simulink model "Boost_FLC_Current_State_Control"  (R2015b)
settings: Solver=ode23t  SolverMode=SingleTasking  StartTime=0.0  StopTime=0.1  FixedStep=1e-8  MinStep=1e-8  RelTol=1e-8
libraries: powerlib x8, fuzblock x2, powerlib_meascontrol x1
settings Model: Creator=Nady  LastModifiedBy=Nady
settings SolverCC: MaxConsecutiveMinStep=10  ZeroCrossAlgorithm=Adaptive  AlgebraicLoopSolver=LineSearch

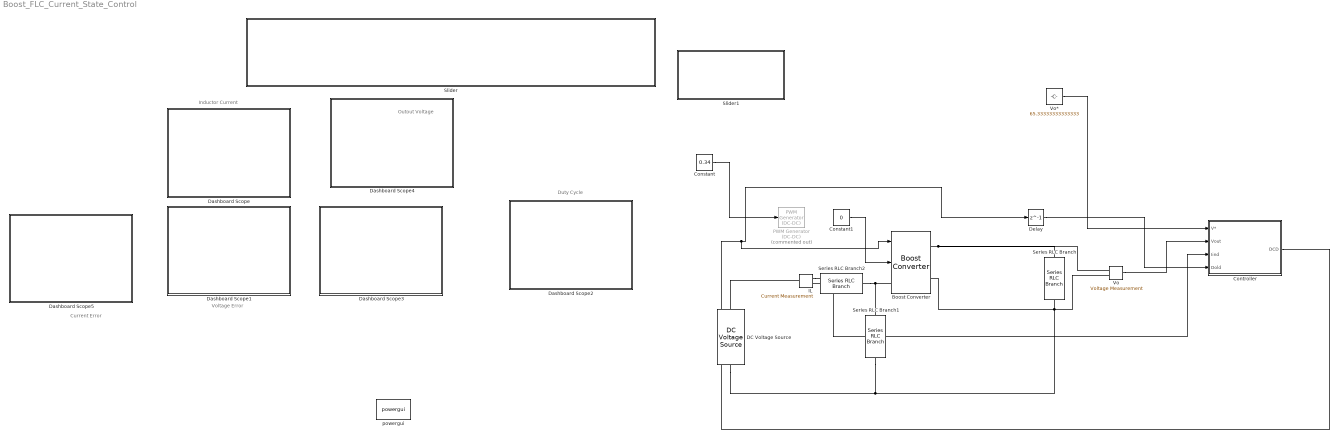
== system Boost_FLC_Current_State_Control ==
  note: Outout Voltage
  note: Inductor Current
  note: Current Error
  note: Duty Cycle
  note: Voltage Error
  Boost Converter : powerlib/Power Electronics/Boost Converter  ModelType=Average model (D-controlled)  Ron=1e-3  Rs=1e6  Cs=inf  Vforward=[0,0]  Ron_Diode=1e-3  Rs_Diode=1e6  Cs_Diode=inf  Vf_Diode=1e-3  Rs_CurrentSource=inf
  Constant : Constant  Value=0.34
  Constant1 : Constant  Value=0
  Controller : Subsystem  TreatAsAtomicUnit=on
  DC Voltage Source : powerlib/Electrical Sources/DC Voltage Source  Amplitude=50  Measurements=None
  Dashboard Scope : Subsystem  DialogController=hmiCreateDDGDialog  IsWebBlock=on  mask(MWDashboardBlock){webBlockId=b3b1b5ba-4a8f-4f28-bbe0-cb5b525e21d4, webBlockType=sdiscope, ShowInitialText=on, HMISrcModelName=Pilot_2_Sub_v4}
      mask prompts: webBlockId "WebBlock Id"; webBlockType "WebBlock Type"; HMISrcModelName "Source Model"
      mask Help: helpview([docroot '/mapfiles/simulink.map'], 'hmi_scope')
      mask Display:
      | if strcmp(get_param(bdroot(gcb),'BlockDiagramType'), 'library')
      |     image([(matlabroot) '/toolbox/simulink/hmi/icons/DashboardScope.png']);
      | end
  Dashboard Scope1 : Subsystem  DialogController=hmiCreateDDGDialog  IsWebBlock=on  mask(MWDashboardBlock){webBlockId=48ecfed1-8b3c-48bc-b34f-bf7039167704, webBlockType=sdiscope, ShowInitialText=on, HMISrcModelName=Pilot_2_Sub_v4}
      mask prompts: webBlockId "WebBlock Id"; webBlockType "WebBlock Type"; HMISrcModelName "Source Model"
      mask Help: helpview([docroot '/mapfiles/simulink.map'], 'hmi_scope')
      mask Display:
      | if strcmp(get_param(bdroot(gcb),'BlockDiagramType'), 'library')
      |     image([(matlabroot) '/toolbox/simulink/hmi/icons/DashboardScope.png']);
      | end
  Dashboard Scope2 : Subsystem  DialogController=hmiCreateDDGDialog  IsWebBlock=on  mask(MWDashboardBlock){webBlockId=b48e5165-dc27-41d1-8306-fea3cbfbff92, webBlockType=sdiscope, ShowInitialText=on, HMISrcModelName=Pilot_2_Sub_v4}
      mask prompts: webBlockId "WebBlock Id"; webBlockType "WebBlock Type"; HMISrcModelName "Source Model"
      mask Help: helpview([docroot '/mapfiles/simulink.map'], 'hmi_scope')
      mask Display:
      | if strcmp(get_param(bdroot(gcb),'BlockDiagramType'), 'library')
      |     image([(matlabroot) '/toolbox/simulink/hmi/icons/DashboardScope.png']);
      | end
  Dashboard Scope3 : Subsystem  DialogController=hmiCreateDDGDialog  IsWebBlock=on  mask(MWDashboardBlock){webBlockId=3429aff5-e82d-44ff-95e7-f1fb18ddd431, webBlockType=sdiscope, ShowInitialText=on, HMISrcModelName=Pilot_2_Sub_v4}
      mask prompts: webBlockId "WebBlock Id"; webBlockType "WebBlock Type"; HMISrcModelName "Source Model"
      mask Help: helpview([docroot '/mapfiles/simulink.map'], 'hmi_scope')
      mask Display:
      | if strcmp(get_param(bdroot(gcb),'BlockDiagramType'), 'library')
      |     image([(matlabroot) '/toolbox/simulink/hmi/icons/DashboardScope.png']);
      | end
  Dashboard Scope4 : Subsystem  DialogController=hmiCreateDDGDialog  IsWebBlock=on  mask(MWDashboardBlock){webBlockId=8e91d4b5-9721-4a03-b8d5-1a874426c786, webBlockType=sdiscope, ShowInitialText=on, HMISrcModelName=Pilot_2_Sub_v4}
      mask prompts: webBlockId "WebBlock Id"; webBlockType "WebBlock Type"; HMISrcModelName "Source Model"
      mask Help: helpview([docroot '/mapfiles/simulink.map'], 'hmi_scope')
      mask Display:
      | if strcmp(get_param(bdroot(gcb),'BlockDiagramType'), 'library')
      |     image([(matlabroot) '/toolbox/simulink/hmi/icons/DashboardScope.png']);
      | end
  Dashboard Scope5 : Subsystem  DialogController=hmiCreateDDGDialog  IsWebBlock=on  mask(MWDashboardBlock){webBlockId=70145929-9d0f-4634-a92b-525ffb0df11a, webBlockType=sdiscope, ShowInitialText=on, HMISrcModelName=Pilot_2_Sub_v4}
      mask prompts: webBlockId "WebBlock Id"; webBlockType "WebBlock Type"; HMISrcModelName "Source Model"
      mask Help: helpview([docroot '/mapfiles/simulink.map'], 'hmi_scope')
      mask Display:
      | if strcmp(get_param(bdroot(gcb),'BlockDiagramType'), 'library')
      |     image([(matlabroot) '/toolbox/simulink/hmi/icons/DashboardScope.png']);
      | end
  Delay : Delay  DelayLength=1  InitialCondition=0  SampleTime=0.0001
  IL : powerlib/Measurements/Current Measurement  PhasorSimulation=off  OutputType=Complex  PSBequivalent=0
  PWM Generator (DC-DC) : powerlib_meascontrol/Pulse & Signal Generators/PWM Generator (DC-DC)  Commented=on  Fsw=5000  Ts=1e-6
  Series RLC Branch : powerlib/Elements/Series RLC Branch  LConnTagsString=__new0  RConnTagsString=__new0  BranchType=RL  Resistance=5000  Inductance=1e-3  SetiL0=off  InitialCurrent=0  Capacitance=1e-6  Setx0=off  InitialVoltage=0  Measurements=None
  Series RLC Branch1 : powerlib/Elements/Series RLC Branch  LConnTagsString=__new0  RConnTagsString=__new0  BranchType=C  Resistance=1  Inductance=1e-3  SetiL0=off  InitialCurrent=0  Capacitance=9e-6  Setx0=off  InitialVoltage=0  Measurements=None
  Series RLC Branch2 : powerlib/Elements/Series RLC Branch  LConnTagsString=__new0  RConnTagsString=__new0  BranchType=R  Resistance=100  Inductance=1e-3  SetiL0=off  InitialCurrent=0  Capacitance=9e-6  Setx0=off  InitialVoltage=0  Measurements=None
  Slider : Subsystem  DialogController=hmiCreateDDGDialog  IsWebBlock=on  mask(MWDashboardBlock){webBlockId=50bee2bc-d1af-434e-aa95-6224faf61a14, webBlockType=slider, ShowInLibBrowser=on, ShowInitialText=on, HMISrcModelName=Pilot_2_Sub_v4}
      mask prompts: webBlockId "WebBlock Id"; webBlockType "WebBlock Type"; HMISrcModelName "Source Model"
      mask Help: helpview([docroot '/mapfiles/simulink.map'], 'hmi_slider')
      mask Display:
      | if strcmp(get_param(bdroot(gcb),'BlockDiagramType'), 'library')
      |     image([(matlabroot) '/toolbox/simulink/hmi/icons/Slider.png']);
      | end
  Slider1 : Subsystem  DialogController=hmiCreateDDGDialog  IsWebBlock=on  mask(MWDashboardBlock){webBlockId=26fbbb97-8c2b-4c3e-8817-68f3be4cb9fd, webBlockType=slider, ShowInLibBrowser=on, ShowInitialText=on, HMISrcModelName=Pilot_2_Sub_v4}
      mask prompts: webBlockId "WebBlock Id"; webBlockType "WebBlock Type"; HMISrcModelName "Source Model"
      mask Help: helpview([docroot '/mapfiles/simulink.map'], 'hmi_slider')
      mask Display:
      | if strcmp(get_param(bdroot(gcb),'BlockDiagramType'), 'library')
      |     image([(matlabroot) '/toolbox/simulink/hmi/icons/Slider.png']);
      | end
  Vo : powerlib/Measurements/Voltage Measurement  PhasorSimulation=off  OutputType=Complex  PSBequivalent=0
  Vo* : Constant  Value=65.33333333333333
  powergui : powerlib/powergui  Priority=1  SimulationMode=Continuous  SolverType=Tustin/Backward Euler (TBE)  SampleTime=1e-6  frequency=60  SPID=off  DisableSnubberDevices=off  DisableRonSwitches=off  DisableVfSwitches=off  SwTol=0  DisplayEquations=off  Interpol=on  ExternalGateDelay=off  methode=off  Ts=10  FunctionMessages=off  echomessages=off  HookPort=off  EnableUseOfTLC=off  x0status=blocks  frequencyindice=0  Pbase=100e6  ErrMax=1e-4  Iterations=50  UnitsV=kV  UnitsW=MW  buscounter=0  RestoreLinks=warning  ResistiveCurrentMeasurement=off  Frange=[0:2:500]  Ylog=off  Xlog=on  ShowGrid=off  save=off  variable=ZData  structure=0  ZoomFFT=off  StartTime=0.0  cycles=1  DisplayStyle=1  fundamental=60  FreqAxis=off  MaxFrequency=1000  frequencyindicesteady=1  RmsSteady=1  display=off
  wires:
  Vo*/1 -> Controller/1(V*)
  Controller/1(DCD) -> Boost Converter/1, Delay/1
  Vo/1 -> Controller/2(Vout)
  IL/1 -> Controller/3(Iind)
  Delay/1 -> Controller/4(Dold)
  Constant/1 -> PWM Generator (DC-DC)/1
  Constant1/1 -> Boost Converter/2
  connections:
  DC Voltage Source/LConn1 -- Series RLC Branch/RConn1 -- Vo/LConn2 -- Boost Converter/RConn2 -- Series RLC Branch1/RConn1
  Boost Converter/RConn1 -- Series RLC Branch/LConn1 -- Vo/LConn1
  Series RLC Branch2/LConn1 -- Series RLC Branch1/LConn1 -- Boost Converter/LConn1
  IL/LConn1 -- DC Voltage Source/RConn1
  Series RLC Branch2/RConn1 -- IL/RConn1

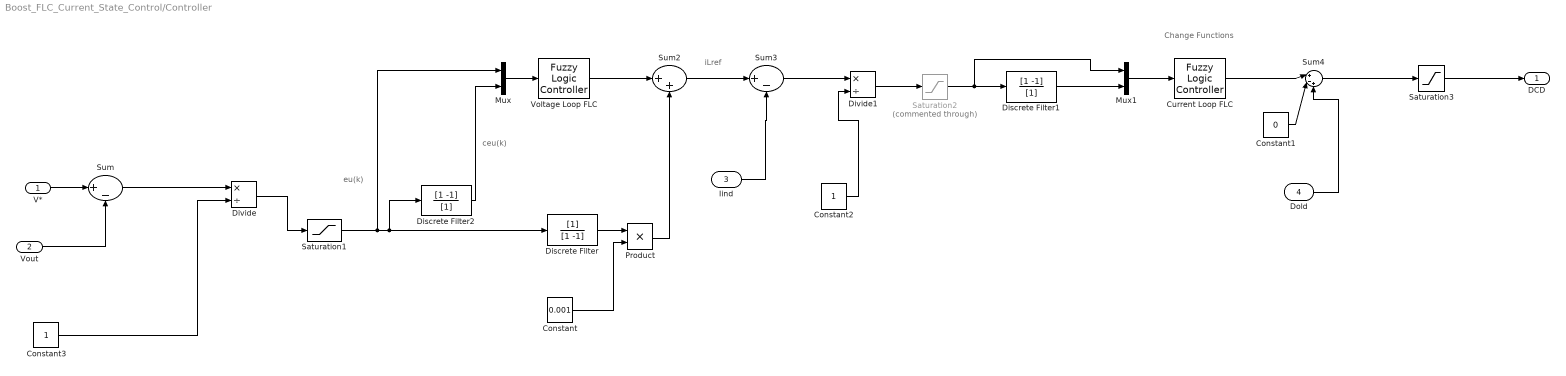
== system Boost_FLC_Current_State_Control/Controller ==
  note: Change Functions
  note: iLref
  note: ceu(k)
  note: eu(k)
  V* : Inport
  Vout : Inport  Port=2
  Iind : Inport  Port=3
  Dold : Inport  Port=4
  Constant : Constant  Value=0.001
  Constant1 : Constant  Value=0  SampleTime=0.0001
  Constant2 : Constant
  Constant3 : Constant
  Current Loop FLC : fuzblock/Fuzzy Logic  Controller  fis=Iloop_v3
  Discrete Filter : DiscreteFilter  Denominator=[1 -1]  SampleTime=0.0001
  Discrete Filter1 : DiscreteFilter  Numerator=[1 -1]  Denominator=[1]  SampleTime=0.0001
  Discrete Filter2 : DiscreteFilter  Numerator=[1 -1]  Denominator=[1]  SampleTime=0.0001
  Divide : Product  Inputs=*/
  Divide1 : Product  Inputs=*/
  Mux : Mux  Inputs=2
  Mux1 : Mux  Inputs=2
  Product : Product
  Saturation1 : Saturate  UpperLimit=70  LowerLimit=-70
  Saturation2 : Saturate  Commented=through  UpperLimit=1  LowerLimit=0
  Saturation3 : Saturate  UpperLimit=0.98  LowerLimit=0
  Sum : Sum  Inputs=|+-
  Sum2 : Sum  Inputs=|++
  Sum3 : Sum  Inputs=|+-
  Sum4 : Sum  Inputs=|+-+
  Voltage Loop FLC : fuzblock/Fuzzy Logic  Controller  fis=Vloop_v3
  DCD : Outport
  wires:
  V*/1 -> Sum/1
  Vout/1 -> Sum/2
  Sum/1 -> Divide/1
  Mux/1 -> Voltage Loop FLC/1
  Voltage Loop FLC/1 -> Sum2/1
  Sum2/1 -> Sum3/1
  Iind/1 -> Sum3/2
  Discrete Filter1/1 -> Mux1/2
  Mux1/1 -> Current Loop FLC/1
  Sum3/1 -> Divide1/1
  Divide1/1 -> Saturation2/1
  Discrete Filter/1 -> Product/1
  Product/1 -> Sum2/2
  Constant/1 -> Product/2
  Current Loop FLC/1 -> Sum4/1
  Constant1/1 -> Sum4/2
  Dold/1 -> Sum4/3
  Constant3/1 -> Divide/2
  Divide/1 -> Saturation1/1
  Constant2/1 -> Divide1/2
  Saturation2/1 -> Mux1/1, Discrete Filter1/1
  Discrete Filter2/1 -> Mux/2
  Saturation1/1 -> Discrete Filter2/1, Discrete Filter/1, Mux/1
  Sum4/1 -> Saturation3/1
  Saturation3/1 -> DCD/1

== system Boost_FLC_Current_State_Control/Dashboard Scope ==

== system Boost_FLC_Current_State_Control/Dashboard Scope1 ==

== system Boost_FLC_Current_State_Control/Dashboard Scope2 ==

== system Boost_FLC_Current_State_Control/Dashboard Scope3 ==

== system Boost_FLC_Current_State_Control/Dashboard Scope4 ==

== system Boost_FLC_Current_State_Control/Dashboard Scope5 ==

== system Boost_FLC_Current_State_Control/Slider ==

== system Boost_FLC_Current_State_Control/Slider1 ==
